simulink model "AM5"  (R2021a)
settings: Solver=VariableStepAuto  StartTime=0.0  StopTime=10.0  RelTol=1e-3
settings Model: Creator=Devraj Kashyap  LastModifiedBy=Devraj Kashyap

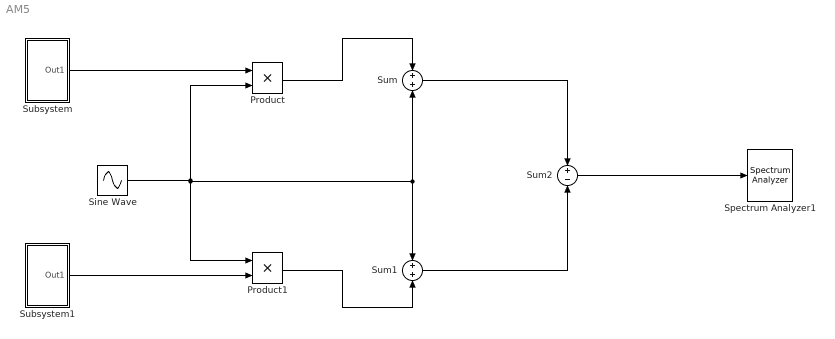
== system AM5 ==
  Product : Product
  Product1 : Product
  Sine Wave : Sin  Amplitude=2  Frequency=100  Phase=90  SampleTime=0.0005
  Spectrum Analyzer1 : SpectrumAnalyzer
  Subsystem : Subsystem
  Subsystem1 : Subsystem
  Sum : Sum  Inputs=+|+
  Sum1 : Sum  Inputs=+|+
  Sum2 : Sum  Inputs=+|-
  wires:
  Sum2/1 -> Spectrum Analyzer1/1
  Subsystem1/1(Out1) -> Product1/2
  Subsystem/1(Out1) -> Product/1
  Sine Wave/1 -> Sum1/1, Sum/2, Product1/1, Product/2
  Product/1 -> Sum/1
  Product1/1 -> Sum1/2
  Sum1/1 -> Sum2/2
  Sum/1 -> Sum2/1

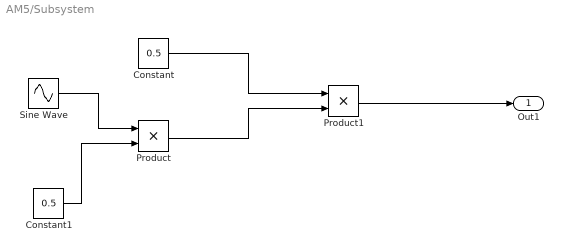
== system AM5/Subsystem ==
  Constant : Constant  Value=0.5  SampleTime=0.0001
  Constant1 : Constant  Value=0.5  SampleTime=0.0005
  Product : Product
  Product1 : Product
  Sine Wave : Sin  Frequency=10  SampleTime=0.0005
  Out1 : Outport
  wires:
  Sine Wave/1 -> Product/1
  Product1/1 -> Out1/1
  Constant1/1 -> Product/2
  Product/1 -> Product1/2
  Constant/1 -> Product1/1

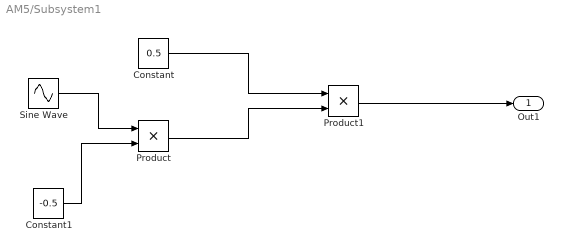
== system AM5/Subsystem1 ==
  Constant : Constant  Value=0.5  SampleTime=0.0001
  Constant1 : Constant  Value=-0.5
  Product : Product
  Product1 : Product
  Sine Wave : Sin  Frequency=10  SampleTime=0.0005
  Out1 : Outport
  wires:
  Sine Wave/1 -> Product/1
  Product1/1 -> Out1/1
  Constant1/1 -> Product/2
  Product/1 -> Product1/2
  Constant/1 -> Product1/1
